simulink model "forward_converter_with_controller"  (R2015a)
settings: Solver=ode45  SolverMode=SingleTasking  StartTime=0.0  StopTime=10.0  MaxStep=1e-4  RelTol=1e-3
libraries: powerlib x13, powerlib_meascontrol x2
settings Model: CovMetricSettings=dwe  CovHtmlReporting=off  covSaveCumulativeToWorkspaceVar=off  CovSaveSingleToWorkspaceVar=off  CovExternalEMLEnable=on  Creator=DELL  LastModifiedBy=DELL
settings DataIOCC: LimitDataPoints=off  SaveFormat=Dataset
settings DebuggingCC: SFUnexpectedBacktrackingDiag=error  SFNoUnconditionalDefaultTransitionDiag=error
settings HardwareCC: ProdBitPerPointer=64  ProdLargestAtomicFloat=Float  ProdIntDivRoundTo=Zero  ProdEndianess=LittleEndian  ProdHWDeviceType=Specified
settings ModelReferenceCC: PropagateSignalLabelsOutOfModel=on
settings GRTTargetCC: TargetLangStandard=C99 (ISO)  GeneratePreprocessorConditionals=Use local settings

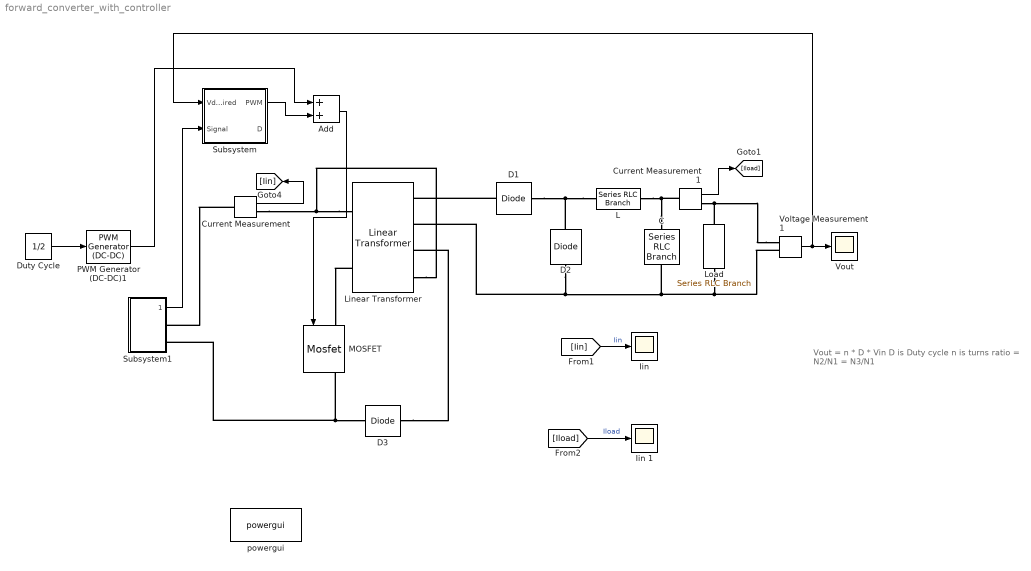
== system forward_converter_with_controller ==
  note: Vout = n * D * Vin
      | D is Duty cycle
      | n is turns ratio = N2/N1 = N3/N1
  Add : Sum
  C : powerlib/Elements/Series RLC Branch  LConnTagsString=__new0  RConnTagsString=__new0  BranchType=C  Resistance=1e-4  Inductance=200e-6  SetiL0=off  InitialCurrent=0  Capacitance=100e-6  Setx0=off  InitialVoltage=0  Measurements=None
  Current Measurement : powerlib/Measurements/Current Measurement  PhasorSimulation=off  OutputType=Complex  PSBequivalent=0
  Current Measurement1 : powerlib/Measurements/Current Measurement  PhasorSimulation=off  OutputType=Complex  PSBequivalent=0
  D1 : powerlib/Power Electronics/Diode  Ron=1e-3  Lon=0  Vf=0  IC=0  UseSnubber=off  Rs=inf  Cs=0  Measurements=off
  D2 : powerlib/Power Electronics/Diode  Ron=1e-3  Lon=0  Vf=0  IC=0  UseSnubber=off  Rs=inf  Cs=0  Measurements=off
  D3 : powerlib/Power Electronics/Diode  Ron=1e-3  Lon=0  Vf=0  IC=0  UseSnubber=off  Rs=inf  Cs=0  Measurements=off
  Duty Cycle : Constant  Value=1/2
  "Iin " : Scope
      settings: TimeRange=auto  MaxDataPoints=5000  SaveToWorkspace=off  YMin=-0.39178  YMax=3.52624  SampleTime=-1
  Iin 1 : Scope
      settings: TimeRange=auto  MaxDataPoints=5000  SaveToWorkspace=off  SaveName=ScopeData2  YMin=-10  YMax=10  SampleTime=-1
  L : powerlib/Elements/Series RLC Branch  LConnTagsString=__new0  RConnTagsString=__new0  BranchType=L  Resistance=10  Inductance=400e-6  SetiL0=off  InitialCurrent=0  Capacitance=400e-6  Setx0=off  InitialVoltage=0  Measurements=Branch current
  Linear Transformer : powerlib/Elements/Linear Transformer  UNITS=SI  NominalPower=[ 250e6 100e3 ]  winding1=[24 0 0]  winding2=[24 0 0]  ThreeWindings=on  winding3=[24 0 0]  RmLm=[1.0805e+06 2866]  Measurements=None  DataType=on
  Load : powerlib/Elements/Series RLC Branch  LConnTagsString=__new0  RConnTagsString=__new0  BranchType=R  Resistance=10  Inductance=200e-6  SetiL0=off  InitialCurrent=0  Capacitance=400e-6  Setx0=off  InitialVoltage=0  Measurements=Branch current
  MOSFET : powerlib/Power Electronics/Mosfet  Ron=1e-3  Lon=0  Rd=1e-3  Vfd=0  IC=0  Rs=1e6  Cs=inf  Measurements=on
  PWM Generator (DC-DC)1 : powerlib_meascontrol/Pulse & Signal Generators/PWM Generator (DC-DC)  Fsw=150e3  Ts=0
  Subsystem : Subsystem
  Subsystem1 : Subsystem
  Voltage Measurement1 : powerlib/Measurements/Voltage Measurement  PhasorSimulation=off  OutputType=Complex  PSBequivalent=0
  "Vout " : Scope
      settings: TimeRange=auto  MaxDataPoints=5000  SaveToWorkspace=off  SaveName=ScopeData  YMin=-2.60677  YMax=23.46089  SampleTime=-1
  powergui : powerlib/powergui  Priority=1  SimulationMode=Continuous  SampleTime=50e-6  frequency=60  Iterations=50  frequencyindice=0  Pbase=100e6  ErrMax=1e-4  UnitsV=kV  UnitsW=MW  buscounter=0  FunctionMessages=off  echomessages=off  EnableUseOfTLC=off  CurrentSourceSwitches=off  DisableSnubberDevices=off  DisableRonSwitches=off  DisableVfSwitches=off  DisplayEquations=off  SolverType=Tustin/Backward Euler (TBE)  Interpol=off  ExternalGateDelay=off  methode=off  Ts=100  x0status=blocks  SPID=on  SwTol=0  HookPort=off  RestoreLinks=warning  ResistiveCurrentMeasurement=off  Frange=[0:2:500]  Ylog=off  Xlog=on  ShowGrid=off  save=off  variable=ZData  structure=0  ZoomFFT=off  StartTime=0.0  cycles=1  DisplayStyle=1  fundamental=60  FreqAxis=off  MaxFrequency=1000  frequencyindicesteady=1  RmsSteady=1  display=off
  wires:
  Duty Cycle/1 -> PWM Generator (DC-DC)1/1
  Current Measurement1/1 -> [Iload]
  [Iload] -> Iin 1/1  "Iload"
  [Iin] -> "Iin "/1  "Iin"
  Current Measurement/1 -> [Iin]
  Subsystem1/1(Signal) -> Subsystem/2(Signal)
  Subsystem/1(PWM) -> Add/2
  PWM Generator (DC-DC)1/1 -> Add/1
  Add/1 -> MOSFET/1
  Voltage Measurement1/1 -> Subsystem/1(Vdesired), "Vout "/1
  connections:
  Voltage Measurement1/LConn2 -- D2/LConn1 -- Linear Transformer/RConn2 -- C/RConn1 -- Load/RConn1
  MOSFET/RConn1 -- Subsystem1/RConn2 -- D3/LConn1
  Voltage Measurement1/LConn1 -- Load/LConn1 -- Current Measurement1/RConn1
  Linear Transformer/LConn1 -- Linear Transformer/RConn4 -- Current Measurement/RConn1
  C/LConn1 -- L/RConn1 -- Current Measurement1/LConn1
  L/LConn1 -- D2/RConn1 -- D1/RConn1
  Linear Transformer/LConn2 -- MOSFET/LConn1
  D3/RConn1 -- Linear Transformer/RConn3
  Current Measurement/LConn1 -- Subsystem1/RConn1
  D1/LConn1 -- Linear Transformer/RConn1

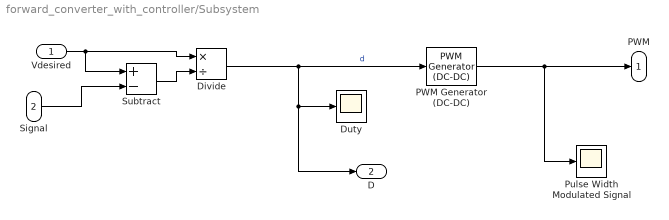
== system forward_converter_with_controller/Subsystem ==
  Vdesired : Inport
  Signal : Inport  Port=2
  Divide : Product  Inputs=*/
  Duty : Scope
      settings: TimeRange=auto  MaxDataPoints=5000  SaveToWorkspace=off  SaveName=ScopeData6  YMin=-0.13346  YMax=0.68158  SampleTime=-1
  PWM Generator (DC-DC) : powerlib_meascontrol/Pulse & Signal Generators/PWM Generator (DC-DC)  Fsw=150e3  Ts=0
  "Pulse Width Modulated Signal " : Scope
      settings: TimeRange=auto  MaxDataPoints=5000  SaveToWorkspace=off  SaveName=ScopeData2  YMin=-0.125  YMax=1.125  SampleTime=-1
  Subtract : Sum  Inputs=+-
  PWM : Outport
  D : Outport  Port=2
  wires:
  PWM Generator (DC-DC)/1 -> "Pulse Width Modulated Signal "/1, PWM/1
  Divide/1 -> PWM Generator (DC-DC)/1, D/1, Duty/1  "d"
  Vdesired/1 -> Subtract/1, Divide/1
  Signal/1 -> Subtract/2
  Subtract/1 -> Divide/2

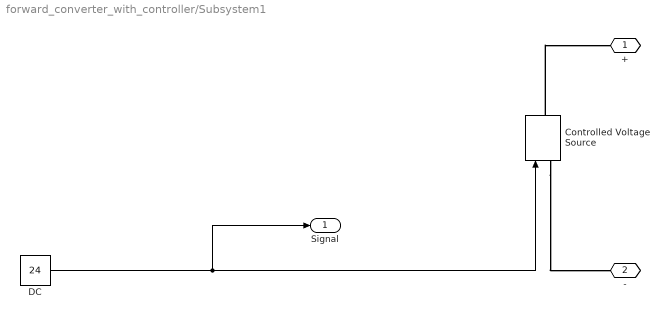
== system forward_converter_with_controller/Subsystem1 ==
  Controlled Voltage Source : powerlib/Electrical Sources/Controlled Voltage Source  Initialize=on  Source_Type=DC  Amplitude=0  Phase=0  Frequency=300  Measurements=None
  DC : Constant  Value=24
  + : PMIOPort  Port=1  Side=Right
  - : PMIOPort  Port=2  Side=Right
  Signal : Outport
  wires:
  DC/1 -> Controlled Voltage Source/1, Signal/1
  connections:
  Controlled Voltage Source/RConn1 -- +/RConn1
  Controlled Voltage Source/LConn1 -- -/RConn1
